simulink model "HIV_model_canon_integral_simulink"  (Simulink 7.5)
settings: Solver=ode3  StartTime=0.0  StopTime=160  FixedStep=0.001  RelTol=1e-3
values from neighbouring files (symbols this model uses):
  sys_big = ss(A_big,B_big,C_big,0)    [HIV_model.m]
settings Model: Creator=Bluecore  LastModifiedBy=michal
settings SolverCC: ShapePreserveControl=EnableAll
settings DebuggingCC: FcnCallInpInsideContextMsg=Enable All

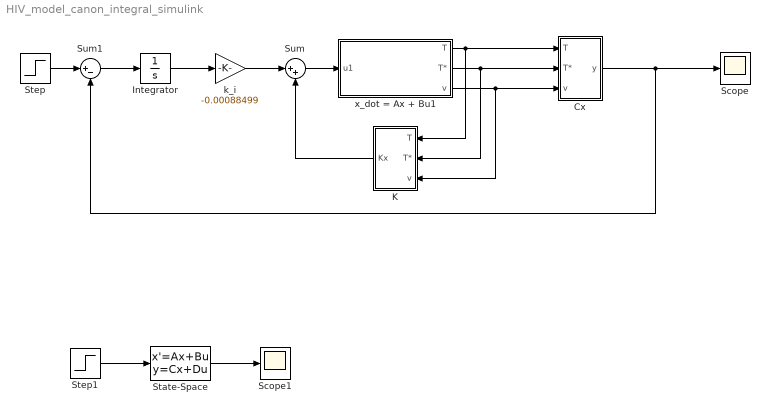
== system HIV_model_canon_integral_simulink ==
  Cx : Subsystem
  Integrator : Integrator
  K : Subsystem
  Scope : Scope
      settings: TimeRange=160  YMin=0  YMax=1.4  SaveName=ScopeData_Integral  DataFormat=Array
  Scope1 : Scope
      settings: TimeRange=160  YMin=0  YMax=1.4  SaveName=ScopeData_Integral1  DataFormat=Array
  State-Space : StateSpace  A=sys_big.a  B=sys_big.b  C=sys_big.c  D=sys_big.d
  Step : Step  Time=0  SampleTime=0
  Step1 : Step  Time=0  SampleTime=0
  Sum : Sum  Inputs=|++
  Sum1 : Sum  Inputs=|+-
  k_i : Gain  Gain=-0.00088499
  x_dot = Ax + Bu1 : Subsystem
  wires:
  Sum/1 -> x_dot = Ax + Bu1/1(u1)
  x_dot = Ax + Bu1/1(T) -> Cx/1(T), K/1(T)
  x_dot = Ax + Bu1/2(T*) -> Cx/2(T*), K/2(T*)
  x_dot = Ax + Bu1/3(v) -> Cx/3(v), K/3(v)
  K/1(Kx) -> Sum/2
  Cx/1(y) -> Sum1/2, Scope/1
  Integrator/1 -> k_i/1
  k_i/1 -> Sum/1
  Step/1 -> Sum1/1
  Sum1/1 -> Integrator/1
  Step1/1 -> State-Space/1
  State-Space/1 -> Scope1/1

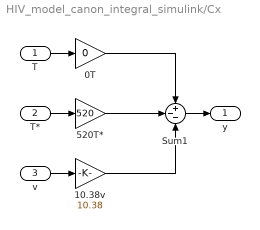
== system HIV_model_canon_integral_simulink/Cx ==
  T : Inport
  T* : Inport  Port=2
  v : Inport  Port=3
  0T : Gain  Gain=0
  10.38v : Gain  Gain=10.38
  520T* : Gain  Gain=520
  Sum1 : Sum  Inputs=+--
  y : Outport
  wires:
  0T/1 -> Sum1/1
  520T*/1 -> Sum1/2
  10.38v/1 -> Sum1/3
  T/1 -> 0T/1
  T*/1 -> 520T*/1
  Sum1/1 -> y/1
  v/1 -> 10.38v/1

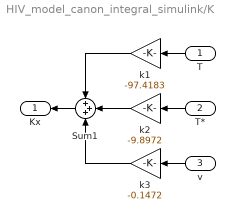
== system HIV_model_canon_integral_simulink/K ==
  T : Inport
  T* : Inport  Port=2
  v : Inport  Port=3
  Sum1 : Sum  Inputs=+++
  k1 : Gain  Gain=-97.4183
  k2 : Gain  Gain=-9.8972
  k3 : Gain  Gain=-0.1472
  Kx : Outport
  wires:
  k1/1 -> Sum1/1
  k2/1 -> Sum1/2
  k3/1 -> Sum1/3
  T/1 -> k1/1
  Sum1/1 -> Kx/1
  T*/1 -> k2/1
  v/1 -> k3/1

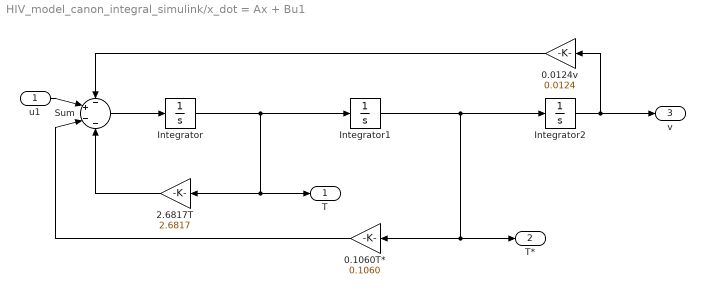
== system HIV_model_canon_integral_simulink/x_dot = Ax + Bu1 ==
  u1 : Inport
  0.0124v : Gain  Gain=0.0124
  0.1060T* : Gain  Gain=0.1060
  2.6817T : Gain  Gain=2.6817
  Integrator : Integrator
  Integrator1 : Integrator
  Integrator2 : Integrator
  Sum : Sum  Inputs=-+--
  T : Outport
  T* : Outport  Port=2
  v : Outport  Port=3
  wires:
  Integrator/1 -> Integrator1/1, 2.6817T/1, T/1
  Integrator1/1 -> Integrator2/1, 0.1060T*/1, T*/1
  Sum/1 -> Integrator/1
  2.6817T/1 -> Sum/4
  0.1060T*/1 -> Sum/3
  Integrator2/1 -> 0.0124v/1, v/1
  0.0124v/1 -> Sum/1
  u1/1 -> Sum/2
